simulink model "NeuronBehaviorTest"  (Simulink 8.4)
settings: Solver=ode45  StartTime=0.0  StopTime=10  RelTol=1e-3
libraries: NeuroModelerLibrary x12
settings Model: Creator=Tim  LastModifiedBy=Tim
settings OptimizationCC: InitFltsAndDblsToZero=on

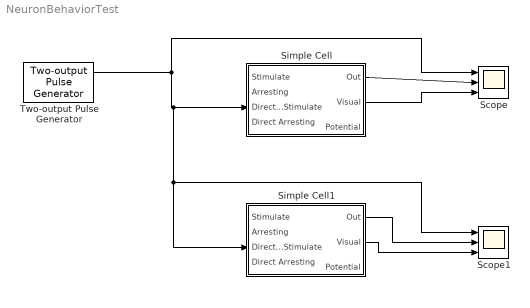
== system NeuronBehaviorTest ==
  Scope : Scope  NumInputPorts=3
      settings: YMin=-1~0~-1  YMax=1~1e-07~0
  Scope1 : Scope  NumInputPorts=3
      settings: YMin=-1~0~-1  YMax=1~1e-07~0
  Simple Cell : Subsystem  AncestorBlock=NeuroModelerLibrary/Simple Cells/Simple Cell
  Simple Cell1 : Subsystem  AncestorBlock=NeuroModelerLibrary/Simple Cells/Simple Cell
  Two-output Pulse Generator : NeuroModelerLibrary/Support/Two-output Pulse Generator  A=0.01  P1=2000  P2=2000  PW=1000  ST=0.001  OOn1=5  OOff1=5.5  OOn2=1.1  OOff2=1.2
  wires:
  Two-output Pulse Generator/1 -> Scope/1, Scope1/1, Simple Cell1/3(Direct Stimulate), Simple Cell/3(Direct Stimulate)
  Simple Cell/1(Out) -> Scope/2
  Simple Cell/2(Visual) -> Scope/3
  Simple Cell1/1(Out) -> Scope1/2
  Simple Cell1/2(Visual) -> Scope1/3

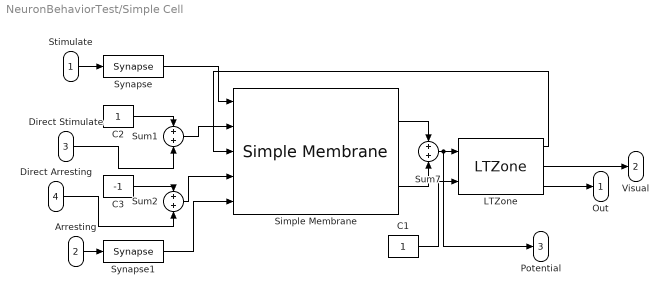
== system NeuronBehaviorTest/Simple Cell ==
  Stimulate : Inport
  Arresting : Inport  Port=2
  Direct Stimulate : Inport  Port=3
  Direct Arresting : Inport  Port=4
  C1 : Constant
  C2 : Constant
  C3 : Constant  Value=-1
  LTZone : NeuroModelerLibrary/Neuron Elements/LTZone  NM=1  FB=1.7  IT=0.005  T=0.001
  Simple Membrane : NeuroModelerLibrary/Neuron Elements/Simple Membrane  ACm=1e-9  ARm=1e7  ECm=1e-9  ERm=1e7  ARFm=1e7  ERFm=1e8
  Sum1 : Sum  SaturateOnIntegerOverflow=on  InputSameDT=on  OutDataTypeStr=Inherit: Same as first input
  Sum2 : Sum  SaturateOnIntegerOverflow=on  InputSameDT=on  OutDataTypeStr=Inherit: Same as first input
  Sum7 : Sum  SaturateOnIntegerOverflow=on  InputSameDT=on  OutDataTypeStr=Inherit: Same as first input
  Synapse : NeuroModelerLibrary/Neuron Elements/Synapse  SecretionTC=0.001  DecompositionTC=0.01  UseKsi=on  ksi=2  gamma=1e8
  Synapse1 : NeuroModelerLibrary/Neuron Elements/Synapse  SecretionTC=0.001  DecompositionTC=0.01  UseKsi=on  ksi=2  gamma=1e8
  Out : Outport
  Visual : Outport  Port=2
  Potential : Outport  Port=3
  wires:
  Synapse1/1 -> Simple Membrane/5
  Synapse/1 -> Simple Membrane/1
  Simple Membrane/2 -> Sum7/2
  Simple Membrane/1 -> Sum7/1
  LTZone/1 -> Simple Membrane/3
  Sum7/1 -> Potential/1, LTZone/1
  Arresting/1 -> Synapse1/1
  Stimulate/1 -> Synapse/1
  C1/1 -> LTZone/2
  LTZone/3 -> Out/1
  LTZone/2 -> Visual/1
  C2/1 -> Sum1/1
  Sum1/1 -> Simple Membrane/2
  Direct Stimulate/1 -> Sum1/2
  Sum2/1 -> Simple Membrane/4
  C3/1 -> Sum2/1
  Direct Arresting/1 -> Sum2/2

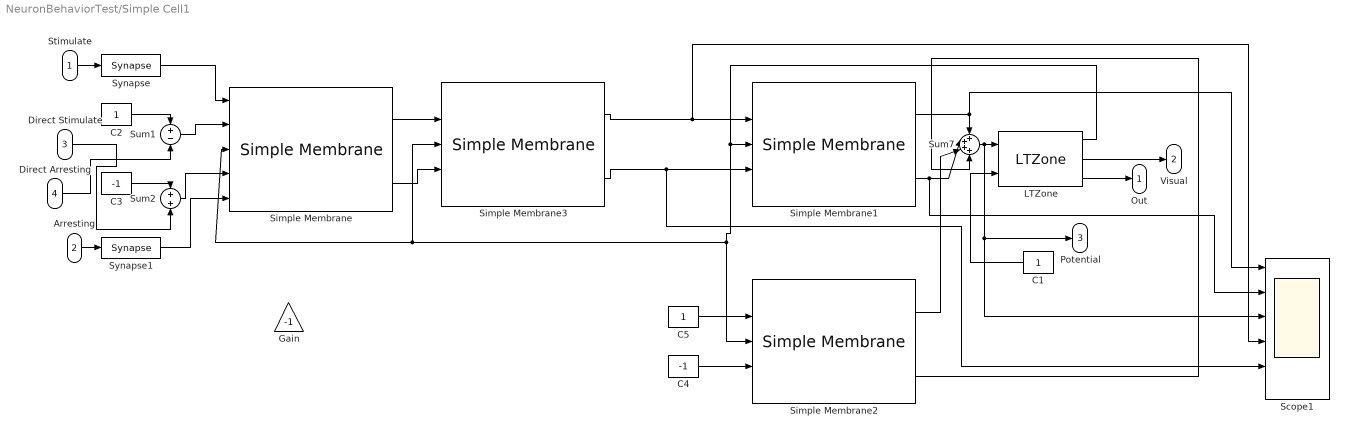
== system NeuronBehaviorTest/Simple Cell1 ==
  Stimulate : Inport
  Arresting : Inport  Port=2
  Direct Stimulate : Inport  Port=3
  Direct Arresting : Inport  Port=4
  C1 : Constant
  C2 : Constant
  C3 : Constant  Value=-1
  C4 : Constant  Value=-1
  C5 : Constant
  Gain : Gain  Gain=-1  SaturateOnIntegerOverflow=on  OutDataTypeStr=Inherit: Same as input  ParamDataTypeStr=Inherit: Same as input
  LTZone : NeuroModelerLibrary/Neuron Elements/LTZone  NM=1  FB=1.7  IT=0.005  T=0.001
  Scope1 : Scope  NumInputPorts=6
      settings: YMin=-1~0~-1~-5~-5~-5  YMax=1~1e-07~0~5~5~5  SaveName=ScopeData2
  Simple Membrane : NeuroModelerLibrary/Neuron Elements/Simple Membrane  ACm=1e-9  ARm=1e7  ECm=1e-9  ERm=1e7  ARFm=1e8  ERFm=1e8
  Simple Membrane1 : NeuroModelerLibrary/Neuron Elements/Simple Membrane  ACm=1e-9  ARm=1e7  ECm=1e-9  ERm=1e7  ARFm=1e8  ERFm=1e8
  Simple Membrane2 : NeuroModelerLibrary/Neuron Elements/Simple Membrane  ACm=1e-9  ARm=1e7  ECm=1e-9  ERm=1e7  ARFm=1e8  ERFm=1e8
  Simple Membrane3 : NeuroModelerLibrary/Neuron Elements/Simple Membrane  ACm=1e-9  ARm=1e9  ECm=1e-9  ERm=1e9  ARFm=1e7  ERFm=1e8
  Sum1 : Sum  Inputs=+-  SaturateOnIntegerOverflow=on  InputSameDT=on  OutDataTypeStr=Inherit: Same as first input
  Sum2 : Sum  SaturateOnIntegerOverflow=on  InputSameDT=on  OutDataTypeStr=Inherit: Same as first input
  Sum7 : Sum  Inputs=++++  SaturateOnIntegerOverflow=on  InputSameDT=on  OutDataTypeStr=Inherit: Same as first input
  Synapse : NeuroModelerLibrary/Neuron Elements/Synapse  SecretionTC=0.001  DecompositionTC=0.01  UseKsi=on  ksi=2  gamma=1e8
  Synapse1 : NeuroModelerLibrary/Neuron Elements/Synapse  SecretionTC=0.001  DecompositionTC=0.01  UseKsi=on  ksi=2  gamma=1e8
  Out : Outport
  Visual : Outport  Port=2
  Potential : Outport  Port=3
  wires:
  Synapse1/1 -> Simple Membrane/5
  Synapse/1 -> Simple Membrane/1
  Sum7/1 -> Scope1/3, Potential/1, LTZone/1
  Arresting/1 -> Synapse1/1
  Stimulate/1 -> Synapse/1
  C1/1 -> LTZone/2
  LTZone/3 -> Out/1
  LTZone/2 -> Visual/1
  C2/1 -> Sum1/1
  Sum1/1 -> Simple Membrane/2
  Direct Stimulate/1 -> Sum2/2
  Sum2/1 -> Simple Membrane/4
  C3/1 -> Sum2/1
  Simple Membrane3/1 -> Scope1/4, Simple Membrane1/2
  Simple Membrane3/2 -> Scope1/5, Simple Membrane1/4
  Simple Membrane1/1 -> Scope1/1, Sum7/1
  Simple Membrane1/2 -> Scope1/2, Sum7/2
  Simple Membrane2/1 -> Sum7/3
  Simple Membrane2/2 -> Sum7/4
  C5/1 -> Simple Membrane2/2
  C4/1 -> Simple Membrane2/4
  Simple Membrane/1 -> Simple Membrane3/2
  Simple Membrane/2 -> Simple Membrane3/4
  Direct Arresting/1 -> Sum1/2
  LTZone/1 -> Simple Membrane3/3, Simple Membrane/3, Simple Membrane2/3, Simple Membrane1/3
